simulink model "PLL2_Analog"  (R2019b)
settings: Solver=ode23  StartTime=0.0  StopTime=tstop  RelTol=1e-5
values from neighbouring files (symbols this model uses):
  dw = 0.1    [LAB2_script.m]
  Kvco = 1    [LAB2_script.m]
  tau = 0.5    [LAB2_script.m]
  w0 = 1e3    (= 1000)    [LAB2_script.m]
  wfr = w0    (= 1000)    [LAB2_script.m]
settings Model: Creator=franc  LastModifiedBy=franc

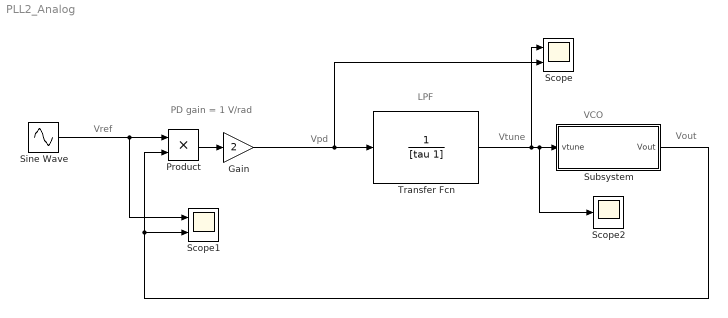
== system PLL2_Analog ==
  note: Vpd
  note: Vtune
  note: Vout
  note: Vref
  note: LPF
  note: VCO
  note: PD gain = 1 V/rad
  Gain : Gain  Gain=2
  Product : Product
  Scope : Scope  NumInputPorts=2
  Scope1 : Scope  NumInputPorts=2
  Scope2 : Scope
  Sine Wave : Sin  Frequency=w0 + dw  SampleTime=0
  Subsystem : Subsystem
  Transfer Fcn : TransferFcn  Denominator=[tau 1]
  wires:
  Sine Wave/1 -> Scope1/1, Product/1
  Product/1 -> Gain/1
  Gain/1 -> Scope/2, Transfer Fcn/1
  Subsystem/1(Vout) -> Scope1/2, Product/2
  Transfer Fcn/1 -> Scope/1, Scope2/1, Subsystem/1(vtune)

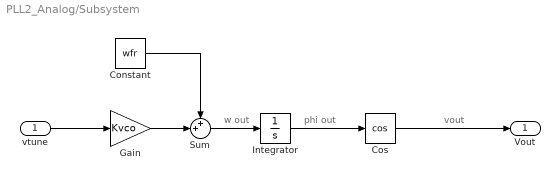
== system PLL2_Analog/Subsystem ==
  note: vout
  note: phi out
  note: w out
  vtune : Inport
  Constant : Constant  Value=wfr
  Cos : Trigonometry  Operator=cos
  Gain : Gain  Gain=Kvco
  Integrator : Integrator
  Sum : Sum  Inputs=++|
  Vout : Outport
  wires:
  vtune/1 -> Gain/1
  Gain/1 -> Sum/2
  Constant/1 -> Sum/1
  Sum/1 -> Integrator/1
  Integrator/1 -> Cos/1
  Cos/1 -> Vout/1
